simulink model "usbSerialLoopBack_Test"  (R2025b)
settings: Solver=FixedStepDiscrete  StartTime=0.0  StopTime=Inf  FixedStep=0.01  RelTol=1e-3  EnableMultiTasking=on
libraries: MagLevTbx_BaseLib x2
settings Model: ExtModeTrigDuration=2  Creator=riccardo  LastModifiedBy=riccardo
settings SolverCC: AutoInsertRateTranBlk=on
settings OptimizationCC: EnhancedBackFolding=on  PassReuseOutputArgsAs=Individual arguments  ZeroExternalMemoryAtStartup=off  ZeroInternalMemoryAtStartup=off  MaxStackSize=64  OptimizeBlockOrder=speed  DifferentSizesBufferReuse=on  OptimizationCustomize=off  EfficientTunableParamExpr=on
settings DebuggingCC: ParameterTunabilityLossMsg=error
settings HardwareCC: ProdBitPerPointer=32.0  ProdBitPerSizeT=32.0  ProdBitPerPtrDiffT=32.0  ProdLargestAtomicInteger=Long  ProdLargestAtomicFloat=Double  ProdWordSize=32.0  ProdHWDeviceType=ARM Compatible->ARM Cortex
settings SFSimCC: MATLABDynamicMemAlloc=off
settings RTWCC: SystemTargetFile=ert.tlc  HardwareBoard=Teensy 4.1 (Arduino Compatible)  TemplateMakefile=ert_default_tmf  Toolchain=Arduino ARM M7  BuildConfiguration=Faster Runs  Description=Embedded Coder
settings CodeAppCC: ForceParamTrailComments=on  IgnoreCustomStorageClasses=off  OperatorAnnotations=on  SimulinkDataObjDesc=on  SFDataObjDesc=on  InsertBlockDesc=on
settings ERTTargetCC: ExtModeTransport=3.0  ExtModeStaticAlloc=on  ExtModeAutomaticAllocSize=off  ExtModeStaticAllocSize=65536.0  ExtModeMexFile=ext_xcp  ExtModeIntrfLevel=Level2 - Open  InlinedParameterPlacement=Hierarchical  RootIOFormat=Structure reference  TargetLangStandard=C99 (ISO)  SupportContinuousTime=on  SupportVariableSizeSignals=on

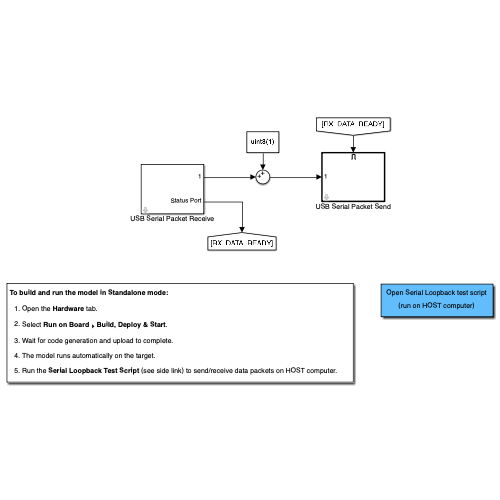
[thumbnail: Simulink's stored preview of the top-level diagram]
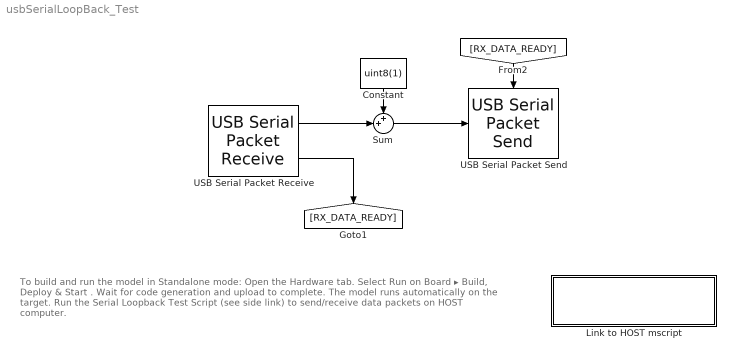
== system usbSerialLoopBack_Test ==
  note: To build and run the model in Standalone mode:
      | Open the Hardware tab.
      | Select Run on Board ▸ Build, Deploy & Start .
      | Wait for code generation and upload to complete.
      | The model runs automatically on the target.
      | Run the Serial Loopback Test Script (see side link) to send/receive data packets on HOST computer.
  Constant : Constant  Value=uint8(1)
  Link to HOST mscript : Subsystem
      settings: OpenFcn=|
      | %  get toolbox base dir
      | info = MagLevTbx_Info();
      | 
      | %  path to HOST matlab script
      | mscriptpath = fullfile( ...
      | info.rootDir, ...
      | 'Examples', ...
      | 'UsbSerialLoopBack_Test', ...
      | 'usbSerialLoopBack_Host'  );
      | 
      | %  open script
      | edit( mscriptpath );
      | 
      | %  clear temp vars
      | clear info mscriptpath;
      mask Display:
      | disp(['Open Serial Loopback test script\n\n' ...
      |     '(run on HOST computer)'])
  Sum : Sum  Inputs=++|
  USB Serial Packet Receive : MagLevTbx_BaseLib/Communication/USB Serial Packet Receive  outputMode=HOLD Outputs  showStatusPort=on  packetSpec={'uint8'}  cobsEncoded=on  nullTerminated=on  sampleTime=-1  showEnablePort=off
      settings: SourceProductName=MagLev Toolbox
  USB Serial Packet Send : MagLevTbx_BaseLib/Communication/USB Serial Packet Send  waitDTR=off  packetSpec={'uint8'}  cobsEncoded=on  nullTerminated=on  sampleTime=-1  showEnablePort=on
      settings: SourceProductName=MagLev Toolbox
  wires:
  USB Serial Packet Receive/2 -> [RX_DATA_READY]
  Constant/1 -> Sum/1
  USB Serial Packet Receive/1 -> Sum/2
  [RX_DATA_READY] -> USB Serial Packet Send/Enable
  Sum/1 -> USB Serial Packet Send/1

== system usbSerialLoopBack_Test/Link to HOST mscript ==
